simulink model "Closed_servo_Observ_for_image"  (R2017a)
settings: Solver=VariableStepAuto  StartTime=0.0  StopTime=10.0  RelTol=1e-3
values from neighbouring files (symbols this model uses):
  A = [A11 A12; A21 A22]    [buck_boost_sys_define.m]
  AObs = A-L*C    [make_graphs.m]    (also in servo_observ.m)
  B = [(Vin+X2)/L; -X1/C]    [buck_boost_sys_define.m]
  BObs = [B , L]    [make_graphs.m]    (also in servo_observ.m)
  C = [0 1]    [buck_boost_sys_define.m]
  CObs = eye(2)    [make_graphs.m]    (also in servo_observ.m)
  D = [0]    [buck_boost_sys_define.m]
  DObs = zeros(2,2)    [make_graphs.m]    (also in servo_observ.m)
  K = Ksrv(j,1:2)    [make_graphs.m]    (also in servo_observ.m = Ksrv(1:2))
  ki = - Ksrv(j,3)    [make_graphs.m]    (also in servo_observ.m = - Ksrv(3))
  U = 0.5    [buck_boost_sys_define.m]
  x0 = [0 0]'    [make_graphs.m]    (also in servo_observ.m)
  x0_hat = [0, 0]'    [make_graphs.m]    (also in servo_observ.m)
libraries: simulink x1
settings Model: Creator=loreliegordon  LastModifiedBy=loreliegordon

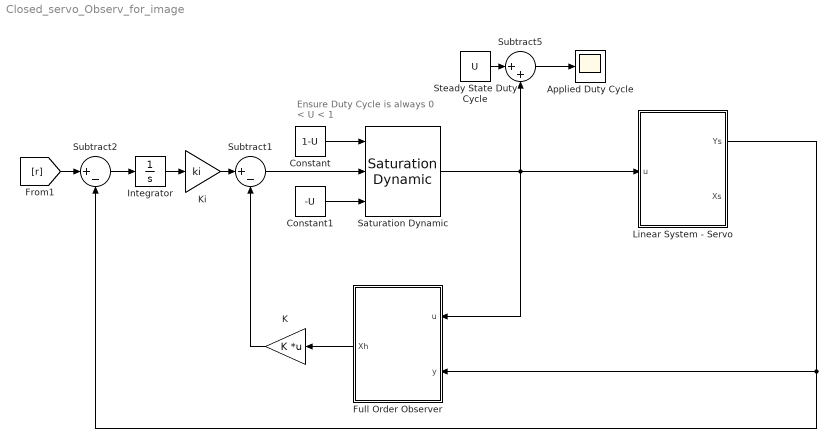
== system Closed_servo_Observ_for_image ==
  note: Ensure Duty Cycle is always
      | 0 < U < 1
  Applied Duty Cycle : Scope
  Constant : Constant  Value=1-U
  Constant1 : Constant  Value=-U
  Full Order Observer : Subsystem
  Integrator : Integrator  InitialCondition=C*x0
  K : Gain  Gain=K  Multiplication=Matrix(K*u) (u vector)
  Ki : Gain  Gain=ki
  Linear System - Servo : Subsystem
  Saturation Dynamic : simulink/Discontinuities/Saturation Dynamic  OutMin=[]  OutMax=[]  OutDataTypeStr=Inherit: Same as second input  OutDataType=fixdt(1, 16)  OutScaling=2^-10  DoSatur=off
  Steady State Duty Cycle : Constant  Value=U
  Subtract1 : Sum  Inputs=|+-
  Subtract2 : Sum  Inputs=|+-
  Subtract5 : Sum  Inputs=|++
  wires:
  Full Order Observer/1(Xh) -> K/1
  Saturation Dynamic/1 -> Linear System - Servo/1(u), Full Order Observer/1(u), Subtract5/2
  Subtract1/1 -> Saturation Dynamic/2
  Steady State Duty Cycle/1 -> Subtract5/1
  Subtract2/1 -> Integrator/1
  Ki/1 -> Subtract1/1
  Subtract5/1 -> Applied Duty Cycle/1
  Linear System - Servo/1(Ys) -> Subtract2/2, Full Order Observer/2(y)
  K/1 -> Subtract1/2
  Integrator/1 -> Ki/1
  Constant/1 -> Saturation Dynamic/1
  Constant1/1 -> Saturation Dynamic/3
  [r] -> Subtract2/1

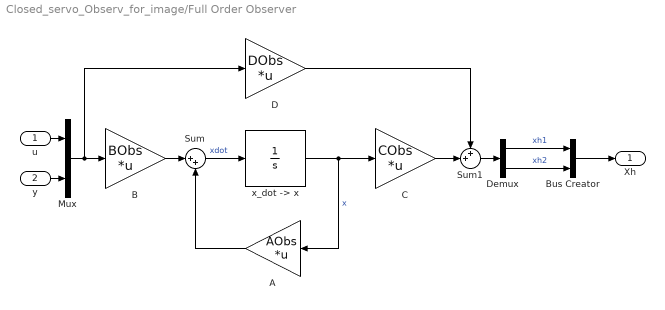
== system Closed_servo_Observ_for_image/Full Order Observer ==
  u : Inport
  y : Inport  Port=2
  A : Gain  Gain=AObs  Multiplication=Matrix(K*u) (u vector)
  B : Gain  Gain=BObs  Multiplication=Matrix(K*u) (u vector)
  Bus Creator : BusCreator  Inputs=2
  C : Gain  Gain=CObs  Multiplication=Matrix(K*u) (u vector)
  D : Gain  Gain=DObs  Multiplication=Matrix(K*u) (u vector)
  Demux : Demux  Outputs=2
  Mux : Mux  Inputs=2
  Sum : Sum  Inputs=|++
  Sum1 : Sum  Inputs=++|
  "x_dot -> x" : Integrator  InitialCondition=x0_hat
  Xh : Outport
  wires:
  Sum/1 -> "x_dot -> x"/1  "xdot"
  "x_dot -> x"/1 -> A/1, C/1  "x"
  A/1 -> Sum/2
  B/1 -> Sum/1
  Mux/1 -> D/1, B/1
  C/1 -> Sum1/2
  D/1 -> Sum1/1
  Demux/1 -> Bus Creator/1  "xh1"
  Demux/2 -> Bus Creator/2  "xh2"
  Bus Creator/1 -> Xh/1
  u/1 -> Mux/1
  y/1 -> Mux/2
  Sum1/1 -> Demux/1

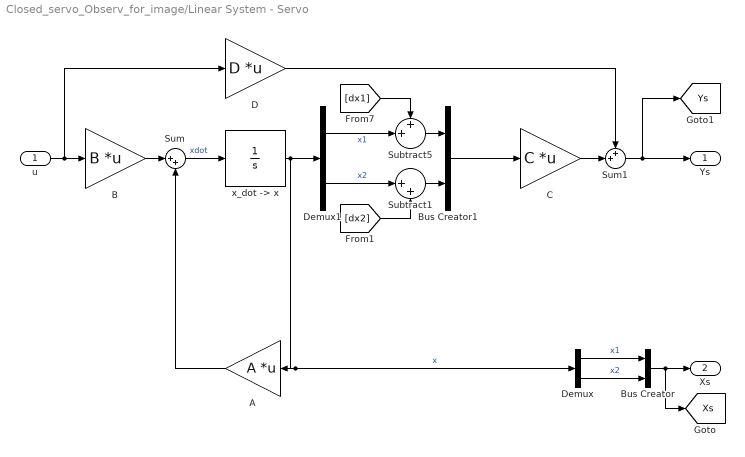
== system Closed_servo_Observ_for_image/Linear System - Servo ==
  u : Inport
  A : Gain  Gain=A  Multiplication=Matrix(K*u) (u vector)
  B : Gain  Gain=B  Multiplication=Matrix(K*u) (u vector)
  Bus Creator : BusCreator  Inputs=2
  Bus Creator1 : BusCreator  Inputs=2
  C : Gain  Gain=C  Multiplication=Matrix(K*u) (u vector)
  D : Gain  Gain=D  Multiplication=Matrix(K*u) (u vector)
  Demux : Demux  Outputs=2
  Demux1 : Demux  Outputs=2
  Subtract1 : Sum  Inputs=|++
  Subtract5 : Sum  Inputs=++|
  Sum : Sum  Inputs=|++
  Sum1 : Sum  Inputs=++|
  "x_dot -> x" : Integrator  InitialCondition=x0
  Ys : Outport
  Xs : Outport  Port=2
  tag scope: Xs=global, Ys=global
  wires:
  Bus Creator/1 -> [Xs], Xs/1
  Demux/2 -> Bus Creator/2  "x2"
  Demux/1 -> Bus Creator/1  "x1"
  Sum1/1 -> Ys/1, [Ys]
  D/1 -> Sum1/1
  C/1 -> Sum1/2
  u/1 -> B/1, D/1
  B/1 -> Sum/1
  A/1 -> Sum/2
  "x_dot -> x"/1 -> Demux/1, A/1, Demux1/1  "x"
  Sum/1 -> "x_dot -> x"/1  "xdot"
  [dx1] -> Subtract5/1
  Demux1/1 -> Subtract5/2  "x1"
  Bus Creator1/1 -> C/1
  Subtract5/1 -> Bus Creator1/1
  Subtract1/1 -> Bus Creator1/2
  Demux1/2 -> Subtract1/1  "x2"
  [dx2] -> Subtract1/2
